simulink model "sf_while"  (Simulink 6.0)
settings: Solver=FixedStepDiscrete  StartTime=0.0  StopTime=1  FixedStep=1  RelTol=1e-3
settings Model: CovMetricSettings=dcmtr  Creator=The MathWorks Inc.  LastModifiedBy=batserve  ExtModeAutoUpdateStatusClock=off
settings DataIOCC: SignalLoggingName=sigsOut
settings DebuggingCC: CheckExecutionContextPreStartOutputMsg=on  CheckExecutionContextRuntimeOutputMsg=on  SolverPrmCheckMsg=none
settings HardwareCC: TargetUnknown=on

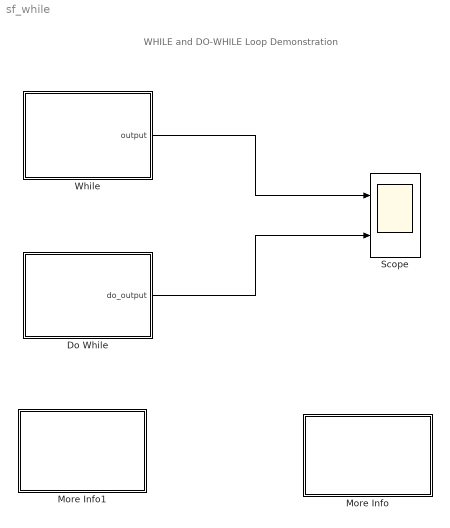
== system sf_while ==
  note: WHILE and DO-WHILE Loop Demonstration
  Do While : Stateflow chart  PropExecContextAcrossSSBoundary=on
  More Info : Subsystem  PropExecContextAcrossSSBoundary=on
      mask Display: disp('Double click\nhere for\ninformation on\nthis demonstration')
  More Info1 : Subsystem  PropExecContextAcrossSSBoundary=on
      settings: OpenFcn=simcad(bdroot);
      mask Display: disp('Double click\nhere for\nSimulink\Stateflow\n Help')
  Scope : Scope  NumInputPorts=2
      settings: TimeRange=1  YMin=0~0  YMax=20~20
  While : Stateflow chart  PropExecContextAcrossSSBoundary=on
  wires:
  Do While/1(do_output) -> Scope/2
  While/1(output) -> Scope/1

== system sf_while/More Info ==
  note: With the use of flow charts, Stateflow allows you to create C-Code or M-Code statements such as
      | the WHILE loop. This particular demo illustrates how a WHILE loop and a DO-WHILE can be
      | implemented in Stateflow in order to create a variable array. The equivalent statements in C-Code
      | are as follows:
      |
      | WHILE:
      | while(condition < 20)
      | {
      |     while_output[i] = condition;
      |     i++;
      |     condition+=2;
      | }
      |
      |
      | DO - WHILE:
      | do
      | {
      |      do_output[i]=condition;
      |      condition+=2;
      |      i++;
      | } while(condition<20);
      |
      | The variable WHILE_OUTPUT is an array with 10 elements and the variable DO_OUTPUT is 11 elements. Notice
      | that in the scope block, the DO-WHILE loops has an extra value of 20 which is what is expected.
      |
      | You can use a such loops to update or buffer a multi-dimensional variable from within Stateflow.
  note: WHILE and DO-WHILE Loop

== system sf_while/More Info1 ==

== stateflow chart While ==
  note: Equivalent C-Code:
      |
      | while(condition < 20)
      | {
      |     while_output[i] = condition;
      |     i++;
      |     condition+=2;
      | }
  (default) -> (junction 4)
  (junction 5) -> (junction 4) : [condition < 20]
      | {while_output[i] =condition;i++;
      | condition+=2;}
  (junction 4) -> (junction 5)
  (junction 5) -> (junction 6) : {output=while_output;}
  data: condition local double; output output double size=[10 1]; i local double; while_output local double size=[10 1]

== stateflow chart Do While ==
  note: Equivalent C-Code
      |
      | do {
      |       do_output[i]=condition;
      |       condition+=2;
      |       i++;
      |      } while(condition<20);
  (default) -> (junction 18)
  (junction 18) -> (junction 19) : {do_output[i]=condition;}
  (junction 19) -> (junction 20) : {do_output;}
  (junction 19) -> (junction 18) : [condition<20]{condition+=2;i++;}
  data: i local double; do_output output double size=[11]; condition local double
